simulink model "Model_visual"  (R2021a)
settings: Solver=VariableStepAuto  StartTime=0.0  StopTime=inf  RelTol=1e-3
undefined symbols (not defined in the file or in its folder): aircraft, FandM, MAV, plotprob, u_trim
settings Model: Creator=DELL  LastModifiedBy=DELL

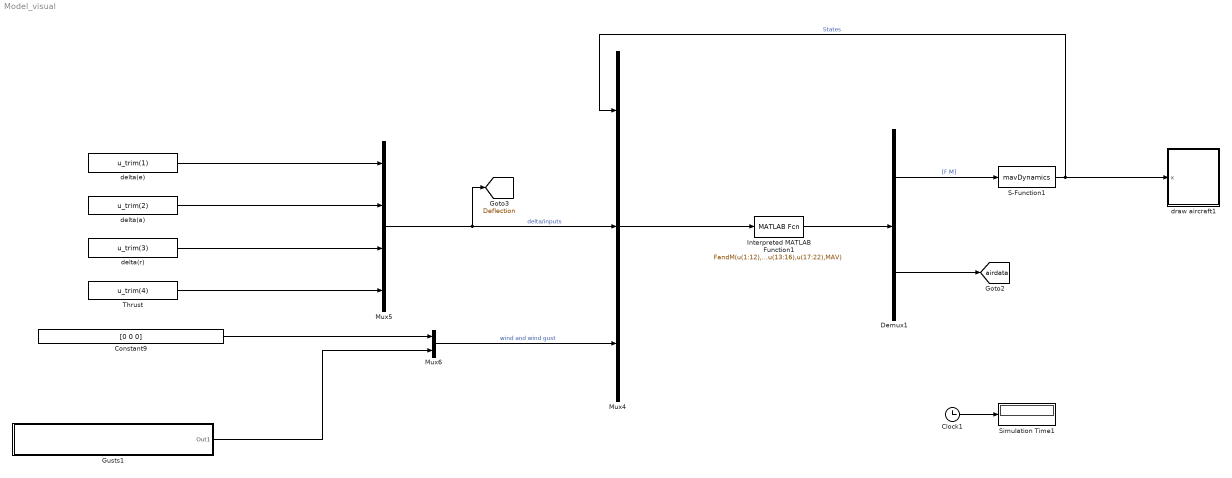
== system Model_visual ==
  Clock1 : Clock
  Constant9 : Constant  Value=[0 0 0]
  Demux1 : Demux  Outputs=[6;6]
  Gusts1 : Subsystem
  Interpreted MATLAB Function1 : MATLABFcn  MATLABFcn=FandM(u(1:12),u(13:16),u(17:22),MAV)  OutputDimensions=12
  Mux4 : Mux  Inputs=3
  Mux5 : Mux
  Mux6 : Mux  Inputs=2
  S-Function1 : S-Function  FunctionName=mavDynamics  Parameters=MAV  SFunctionDeploymentMode=off  EnableBusSupport=off
  Simulation Time1 : Display
  Thrust : Constant  Value=u_trim(4)
  delta(a) : Constant  Value=u_trim(2)
  delta(e) : Constant  Value=u_trim(1)
  delta(r) : Constant  Value=u_trim(3)
  draw aircraft1 : Subsystem
  tag scope: Deflection=global, airdata=global
  wires:
  Mux6/1 -> Mux4/3  "wind and wind gust"
  Demux1/2 -> [airdata]
  Constant9/1 -> Mux6/1
  Mux5/1 -> Mux4/2, [Deflection]  "delta/inputs"
  Clock1/1 -> Simulation Time1/1
  Mux4/1 -> Interpreted MATLAB Function1/1
  Interpreted MATLAB Function1/1 -> Demux1/1
  S-Function1/1 -> draw aircraft1/1(x), Mux4/1  "States"
  Gusts1/1(Out1) -> Mux6/2
  Demux1/1 -> S-Function1/1  "[F M]"
  delta(e)/1 -> Mux5/1
  delta(a)/1 -> Mux5/2
  delta(r)/1 -> Mux5/3
  Thrust/1 -> Mux5/4

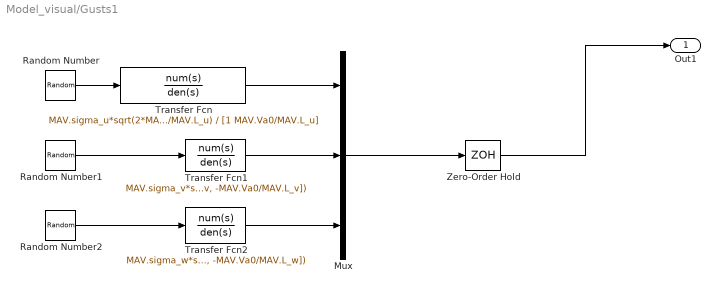
== system Model_visual/Gusts1 ==
  Mux : Mux  Inputs=3
  Random Number : RandomNumber  SampleTime=0.1
  Random Number1 : RandomNumber  SampleTime=0.1
  Random Number2 : RandomNumber  SampleTime=0.1
  Transfer Fcn : TransferFcn  Numerator=MAV.sigma_u*sqrt(2*MAV.Va0/MAV.L_u)  Denominator=[1 MAV.Va0/MAV.L_u]
  Transfer Fcn1 : TransferFcn  Numerator=MAV.sigma_v*sqrt(3*MAV.Va0/MAV.L_u)*[0, 1, MAV.Va0/sqrt(3)/MAV.L_v]  Denominator=poly([-MAV.Va0/MAV.L_v, -MAV.Va0/MAV.L_v])
  Transfer Fcn2 : TransferFcn  Numerator=MAV.sigma_w*sqrt(3*MAV.Va0/MAV.L_u)*[0, 1, MAV.Va0/sqrt(3)/MAV.L_w]  Denominator=poly([-MAV.Va0/MAV.L_w, -MAV.Va0/MAV.L_w])
  Zero-Order Hold : ZeroOrderHold  SampleTime=-1
  Out1 : Outport
  wires:
  Zero-Order Hold/1 -> Out1/1
  Transfer Fcn2/1 -> Mux/3
  Random Number1/1 -> Transfer Fcn1/1
  Transfer Fcn/1 -> Mux/1
  Random Number/1 -> Transfer Fcn/1
  Transfer Fcn1/1 -> Mux/2
  Random Number2/1 -> Transfer Fcn2/1
  Mux/1 -> Zero-Order Hold/1

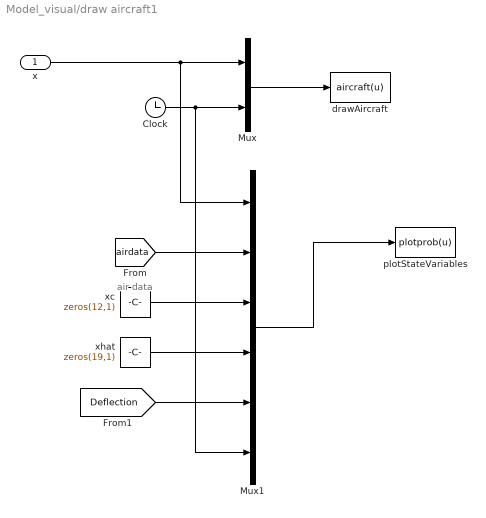
== system Model_visual/draw aircraft1 ==
  note: air data
  x : Inport
  Clock : Clock
  Mux : Mux  Inputs=2
  Mux1 : Mux  Inputs=6
  drawAircraft : MATLABFcn  MATLABFcn=aircraft(u)  OutputDimensions=0  SampleTime=0.1
  plotStateVariables : MATLABFcn  MATLABFcn=plotprob(u)  OutputDimensions=0  SampleTime=0.1
  xc : Constant  Value=zeros(12,1)
  xhat : Constant  Value=zeros(19,1)
  wires:
  [airdata] -> Mux1/2
  [Deflection] -> Mux1/5
  xc/1 -> Mux1/3
  xhat/1 -> Mux1/4
  Mux1/1 -> plotStateVariables/1
  Clock/1 -> Mux1/6, Mux/2
  x/1 -> Mux1/1, Mux/1
  Mux/1 -> drawAircraft/1
